simulink model "validating_low_pass_filter"  (R2012b)
settings: Solver=ode45  StartTime=0.0  StopTime=10/30  FixedStep=1e-5  RelTol=1e-3
values from neighbouring files (symbols this model uses):
  Gd = c2d(G,Ts)    [validating_low_pass_filters.m]
settings Model: Creator=Juliano  LastModifiedBy=Juliano

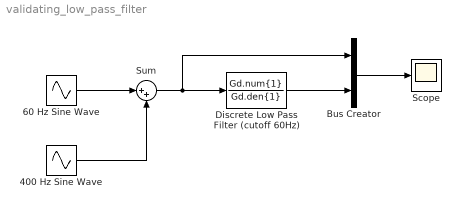
== system validating_low_pass_filter ==
  400 Hz Sine Wave : Sin  Frequency=400*2*pi  SampleTime=0
  60 Hz Sine Wave : Sin  Frequency=30*2*pi  SampleTime=0
  Bus Creator : BusCreator  Inputs=2
  Discrete Low Pass Filter (cutoff 60Hz) : DiscreteTransferFcn  Numerator=Gd.num{1}  Denominator=Gd.den{1}  SampleTime=Gd.Ts
  Scope : Scope
  Sum : Sum  Inputs=|++
  wires:
  Discrete Low Pass Filter (cutoff 60Hz)/1 -> Bus Creator/2
  Bus Creator/1 -> Scope/1
  60 Hz Sine Wave/1 -> Sum/1
  Sum/1 -> Bus Creator/1, Discrete Low Pass Filter (cutoff 60Hz)/1
  400 Hz Sine Wave/1 -> Sum/2
